simulink model "algebraic_equations"  (R2024b)
settings: Solver=VariableStepAuto  StartTime=0.0  StopTime=10.0  RelTol=1e-3
settings Model: Creator=kavin  LastModifiedBy=kavin

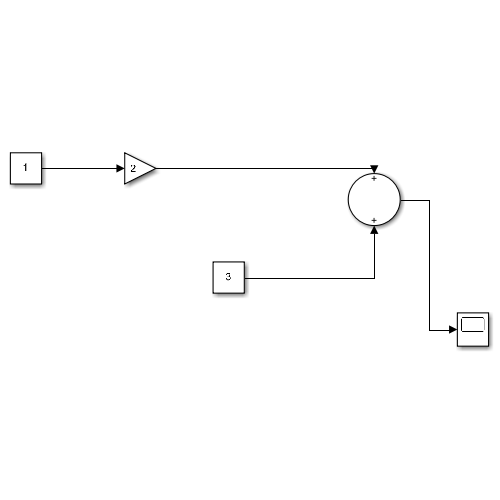
[thumbnail: Simulink's stored preview of the top-level diagram]
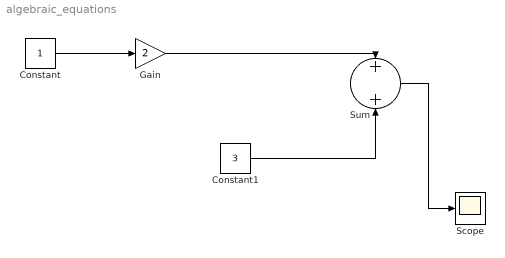
== system algebraic_equations ==
  Constant : Constant
  Constant1 : Constant  Value=3
  Gain : Gain  Gain=2
  Scope : Scope
  Sum : Sum
  wires:
  Sum/1 -> Scope/1
  Constant/1 -> Gain/1
  Gain/1 -> Sum/1
  Constant1/1 -> Sum/2
